simulink model "laghiBrianza"  (Simulink 7.4)
settings: Solver=ode45  StartTime=0.0  StopTime=40  RelTol=1e-3
undefined symbols (not defined in the file): kalserio, kparatie, kpusiano, ksegrino
libraries: simulink x2
settings Model: Creator=DOC_CS31  LastModifiedBy=alessandra
settings DataIOCC: SaveTime=off
settings OptimizationCC: InitFltsAndDblsToZero=on
settings DebuggingCC: SaveWithParameterizedLinksMsg=none
settings GRTTargetCC: TargetFcnLib=ansi_tfl_tmw.mat

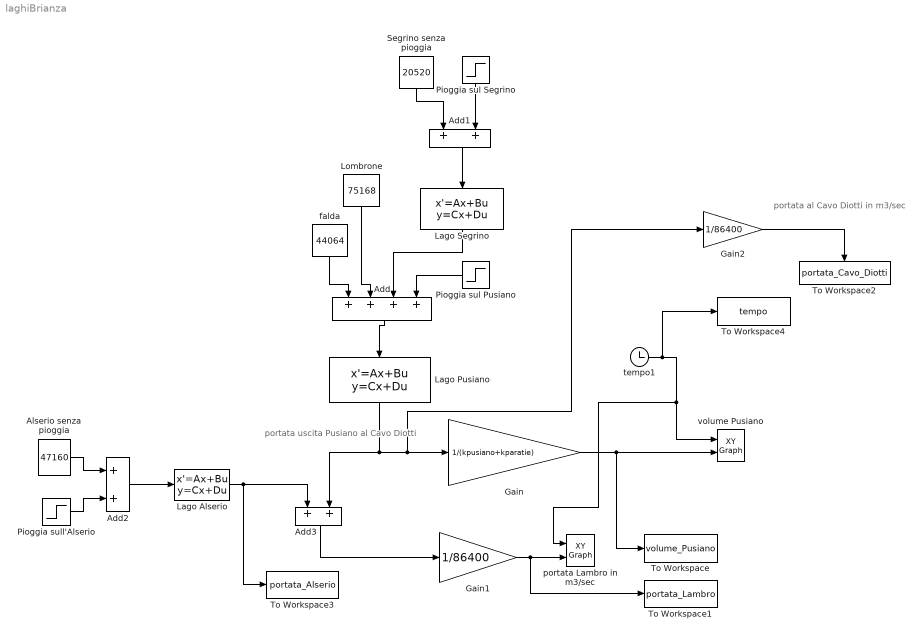
== system laghiBrianza ==
  note: portata uscita
      | Pusiano
      | al Cavo Diotti
  note: portata al Cavo Diotti in m3/sec
  Add : Sum  Inputs=++++  OutDataType=fixdt(1, 16)  OutScaling=2^-10
  Add1 : Sum  OutDataType=fixdt(1, 16)  OutScaling=2^-10
  Add2 : Sum  OutDataType=fixdt(1, 16)  OutScaling=2^-10
  Add3 : Sum  OutDataType=fixdt(1, 16)  OutScaling=2^-10
  Alserio senza pioggia : Constant  Value=47160  OutDataType=fixdt(1, 16)  OutScaling=2^0
  Gain : Gain  Gain=1/(kpusiano+kparatie)  ParameterDataType=fixdt(1, 16)  ParameterScaling=2^0  OutDataType=fixdt(1, 16)  OutScaling=2^0
  Gain1 : Gain  Gain=1/86400  ParameterDataType=fixdt(1, 16)  ParameterScaling=2^0  OutDataType=fixdt(1, 16)  OutScaling=2^0
  Gain2 : Gain  Gain=1/86400  ParameterDataType=fixdt(1, 16)  ParameterScaling=2^0  OutDataType=fixdt(1, 16)  OutScaling=2^0
  Lago Pusiano : StateSpace  A=-kpusiano-kparatie  C=kpusiano+kparatie  D=0  X0=(44064+75168+20520)/(kpusiano)
  Lago Segrino : StateSpace  A=-ksegrino  C=ksegrino  D=0  X0=20520/ksegrino
  Lago Alserio : StateSpace  A=-kalserio  C=kalserio  D=0  X0=47160/kalserio
  Lombrone : Constant  Value=75168  OutDataType=fixdt(1, 16)  OutScaling=2^0
  Pioggia sul Pusiano : Step  Time=10  After=0  SampleTime=0
  Pioggia sul Segrino : Step  Time=10  After=0  SampleTime=0
  Pioggia sull'Alserio : Step  Time=10  After=0  SampleTime=0
  Segrino senza pioggia : Constant  Value=20520  OutDataType=fixdt(1, 16)  OutScaling=2^0
  To Workspace : ToWorkspace  VariableName=volume_Pusiano  SampleTime=-1  SaveFormat=Array
  To Workspace1 : ToWorkspace  VariableName=portata_Lambro  SampleTime=-1  SaveFormat=Array
  To Workspace2 : ToWorkspace  VariableName=portata_Cavo_Diotti  SampleTime=-1  SaveFormat=Array
  To Workspace3 : ToWorkspace  VariableName=portata_Alserio  SampleTime=-1  SaveFormat=Array
  To Workspace4 : ToWorkspace  VariableName=tempo  SampleTime=-1  SaveFormat=Array
  falda : Constant  Value=44064  OutDataType=fixdt(1, 16)  OutScaling=2^0
  portata Lambro in m3/sec : simulink/Sinks/XY Graph  SystemSampleTime=-1  xmin=0  xmax=40  ymin=-1  ymax=8  st=-1
  tempo1 : Clock
      settings: Decimation=10
  volume Pusiano : simulink/Sinks/XY Graph  SystemSampleTime=-1  xmin=0  xmax=40  ymin=-1  ymax=22000000  st=-1
  wires:
  Lombrone/1 -> Add/2
  falda/1 -> Add/1
  Add/1 -> Lago Pusiano/1
  tempo1/1 -> volume Pusiano/1, portata Lambro in m3/sec/1, To Workspace4/1
  Gain/1 -> volume Pusiano/2, To Workspace/1
  Lago Pusiano/1 -> Add3/2, Gain/1, Gain2/1
  Pioggia sul Segrino/1 -> Add1/2
  Segrino senza pioggia/1 -> Add1/1
  Add1/1 -> Lago Segrino/1
  Lago Segrino/1 -> Add/3
  Pioggia sul Pusiano/1 -> Add/4
  Alserio senza pioggia/1 -> Add2/1
  Pioggia sull'Alserio/1 -> Add2/2
  Add2/1 -> Lago Alserio/1
  Lago Alserio/1 -> Add3/1, To Workspace3/1
  Add3/1 -> Gain1/1
  Gain1/1 -> portata Lambro in m3/sec/2, To Workspace1/1
  Gain2/1 -> To Workspace2/1
